simulink subsystem "tehrani_alv_mass_balance_v5"  (R2020b)
settings: Solver=VariableStepAuto  StartTime=0.0  StopTime=10.0  RelTol=1e-3
settings Model: Creator=RH  LastModifiedBy=fonck

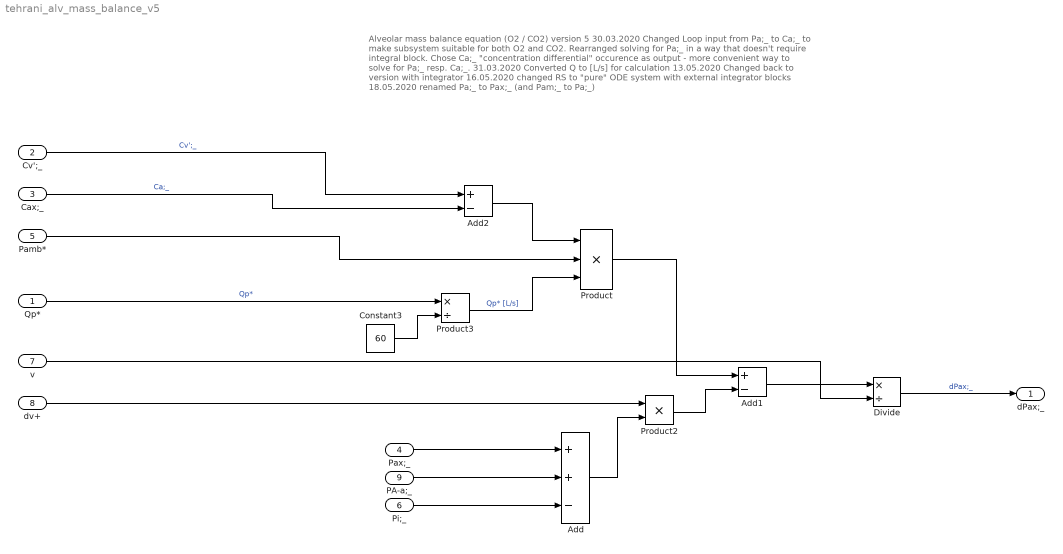
== system tehrani_alv_mass_balance_v5 ==
  note: Alveolar mass balance equation (O2 / CO2) version 5
      |
      | 30.03.2020 Changed Loop input from Pa;_ to Ca;_ to make subsystem suitable for both O2 and CO2.
      | Rearranged solving for Pa;_ in a way that doesn't require integral block.
      | Chose Ca;_ "concentration differential" occurence as output - more convenient way to solve for Pa;_ resp. Ca;_.
      | 31.03.2020 Converted Q to [L/s] for calculation
      | 13.05.2020 Changed back to version with integrator
      | 16.05.2020 changed RS to "pure" ODE system with external integrator blocks
      | 18.05.2020 renamed Pa;_ to Pax;_ (and Pam;_ to Pa;_)
  Qp* : Inport  Unit=L/min
  Cv';_ : Inport  Port=2  Unit=1
  Cax;_ : Inport  Port=3  Unit=1
  Pax;_ : Inport  Port=4  Unit=mmHg
  Pamb* : Inport  Port=5  Unit=mmHg
  Pi;_ : Inport  Port=6  Unit=mmHg
  v : Inport  Port=7  Unit=L
  dv+ : Inport  Port=8  Unit=L/s
  PA-a;_ : Inport  Port=9  Unit=mmHg
  Add : Sum  Inputs=++-
  Add1 : Sum  Inputs=+-
  Add2 : Sum  Inputs=+-
  Constant3 : Constant  Value=60
  Divide : Product  Inputs=*/
  Product : Product  Inputs=***
  Product2 : Product
  Product3 : Product  Inputs=*/
  dPax;_ : Outport  Unit=mmHg/s
  wires:
  Divide/1 -> dPax;_/1  "dPax;_"
  Pax;_/1 -> Add/1
  v/1 -> Divide/2
  Pamb*/1 -> Product/2
  PA-a;_/1 -> Add/2
  Pi;_/1 -> Add/3
  Constant3/1 -> Product3/2
  Product/1 -> Add1/1
  Cv';_/1 -> Add2/1  "Cv';_"
  Product2/1 -> Add1/2
  Product3/1 -> Product/3  "Qp* [L/s]"
  dv+/1 -> Product2/1
  Add/1 -> Product2/2
  Add1/1 -> Divide/1
  Qp*/1 -> Product3/1  "Qp*"
  Add2/1 -> Product/1
  Cax;_/1 -> Add2/2  "Ca;_"
